simulink model "Day04"  (R2024b)
settings: Solver=VariableStepAuto  StartTime=0.0  StopTime=10.0  RelTol=1e-3
settings Model: Creator=jun_mac  LastModifiedBy=jun_mac

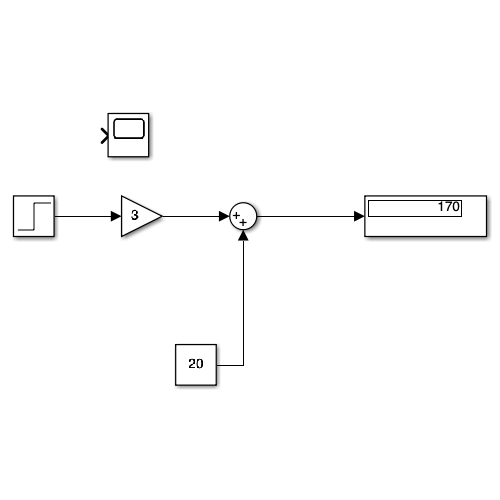
[thumbnail: Simulink's stored preview of the top-level diagram]
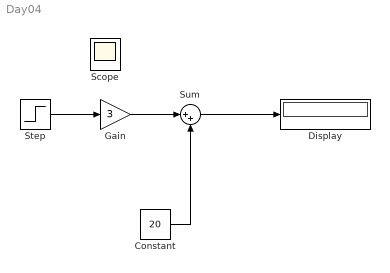
== system Day04 ==
  Constant : Constant  Value=20
  Display : Display
  Gain : Gain  Gain=3
  Scope : Scope
  Step : Step  Time=3  After=50  SampleTime=0
  Sum : Sum  Inputs=|++
  wires:
  Step/1 -> Gain/1
  Sum/1 -> Display/1
  Constant/1 -> Sum/2
  Gain/1 -> Sum/1
